simulink model "clutch_lockup"  (R2020b)
settings: Solver=ode23  StartTime=0.0  StopTime=10.0  RelTol=1e-3
model workspace (MATLAB code in the model file):
  | % Load initial conditions and other information
  | 
  | load sldemo_clutchparam;
undefined symbols (not defined in the file or in its folder): be, bv, Ie, Iv, muk, mus, R
settings Model: DataDictionary=ClutchDataDict.sldd  OrderedModelArguments=off  Creator=DELL  LastModifiedBy=DELL
settings SolverCC: MaxConsecutiveMinStep=5  ZeroCrossAlgorithm=Adaptive
settings DebuggingCC: MaxConsecutiveZCsMsg=none  IgnoredZcDiagnostic=none

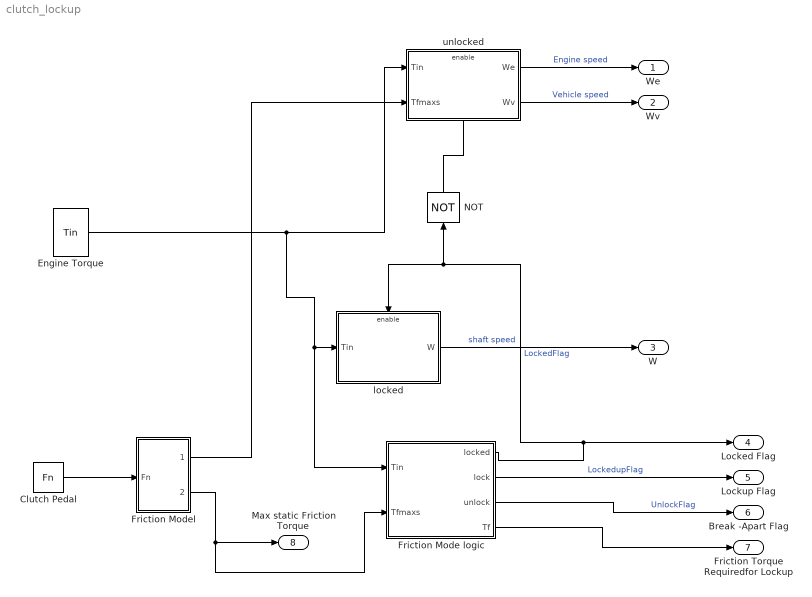
== system clutch_lockup ==
  Clutch Pedal : FromWorkspace  VariableName=Fn  ZeroCross=off
  Engine Torque : FromWorkspace  VariableName=Tin  ZeroCross=off
  Friction Mode logic : Subsystem
  Friction Model : Subsystem
  NOT : Logic  Operator=NOT  IconShape=distinctive  AllPortsSameDT=off  OutDataTypeStr=fixdt(1,16)
  locked : Subsystem
  unlocked : Subsystem
  We : Outport
  Wv : Outport  Port=2
  W : Outport  Port=3
  Locked Flag : Outport  Port=4
  Lockup Flag : Outport  Port=5
  Break -Apart Flag : Outport  Port=6
  Friction Torque Requiredfor Lockup : Outport  Port=7
  Max static Friction Torque : Outport  Port=8
  wires:
  Friction Mode logic/2(lock) -> Lockup Flag/1  "LockedupFlag"
  Friction Mode logic/1(locked) -> Locked Flag/1, NOT/1, locked/Enable  "LockedFlag"
  Friction Model/1(Tfmaxk) -> unlocked/2(Tfmaxs)
  Friction Mode logic/4(Tf) -> Friction Torque Requiredfor Lockup/1
  Friction Mode logic/3(unlock) -> Break -Apart Flag/1  "UnlockFlag"
  Friction Model/2(Tfmaxs) -> Friction Mode logic/2(Tfmaxs), Max static Friction Torque/1
  locked/1(W) -> W/1  "shaft speed"
  NOT/1 -> unlocked/Enable
  Engine Torque/1 -> unlocked/1(Tin), Friction Mode logic/1(Tin), locked/1(Tin)
  unlocked/2(Wv) -> Wv/1  "Vehicle speed"
  unlocked/1(We) -> We/1  "Engine speed"
  Clutch Pedal/1 -> Friction Model/1(Fn)

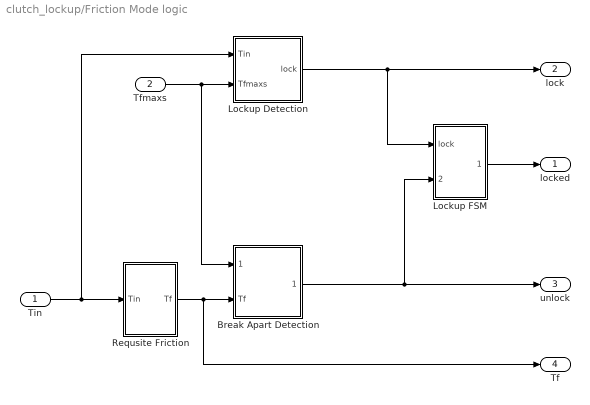
== system clutch_lockup/Friction Mode logic ==
  Tin : Inport
  Tfmaxs : Inport  Port=2
  Break Apart Detection : Subsystem
  Lockup Detection : Subsystem
  Lockup FSM : Subsystem
  Requsite Friction : Subsystem
  locked : Outport
  lock : Outport  Port=2
  unlock : Outport  Port=3
  Tf : Outport  Port=4
  wires:
  Tin/1 -> Lockup Detection/1(Tin), Requsite Friction/1(Tin)
  Requsite Friction/1(Tf) -> Tf/1, Break Apart Detection/2(Tf)
  Tfmaxs/1 -> Break Apart Detection/1(Tfmaxs), Lockup Detection/2(Tfmaxs)
  Lockup FSM/1(locked) -> locked/1
  Lockup Detection/1(lock) -> Lockup FSM/1(lock), lock/1
  Break Apart Detection/1(unlock) -> Lockup FSM/2(unlock), unlock/1

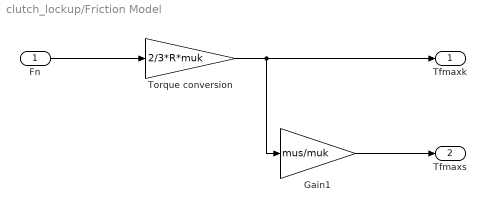
== system clutch_lockup/Friction Model ==
  Fn : Inport
  Gain1 : Gain  Gain=mus/muk
  Torque conversion : Gain  Gain=2/3*R*muk
  Tfmaxk : Outport
  Tfmaxs : Outport  Port=2
  wires:
  Fn/1 -> Torque conversion/1
  Torque conversion/1 -> Gain1/1, Tfmaxk/1
  Gain1/1 -> Tfmaxs/1

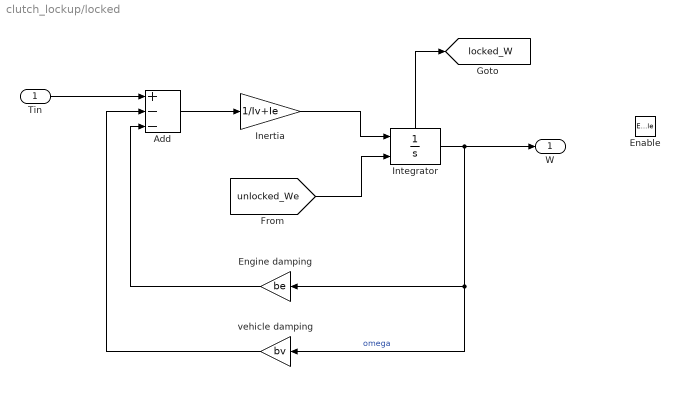
== system clutch_lockup/locked ==
  Tin : Inport
  Enable : EnablePort
  Add : Sum  Inputs=+--
  Engine damping : Gain  Gain=be
  Inertia : Gain  Gain=1/Iv+Ie
  Integrator : Integrator  InitialConditionSource=external  ShowStatePort=on
  vehicle damping : Gain  Gain=bv
  W : Outport
  tag scope: locked_W=global
  wires:
  vehicle damping/1 -> Add/2
  Integrator/1 -> W/1, Engine damping/1, vehicle damping/1  "omega"
  Tin/1 -> Add/1
  Engine damping/1 -> Add/3
  Integrator/State -> [locked_W]
  Inertia/1 -> Integrator/1
  Add/1 -> Inertia/1
  [unlocked_We] -> Integrator/2

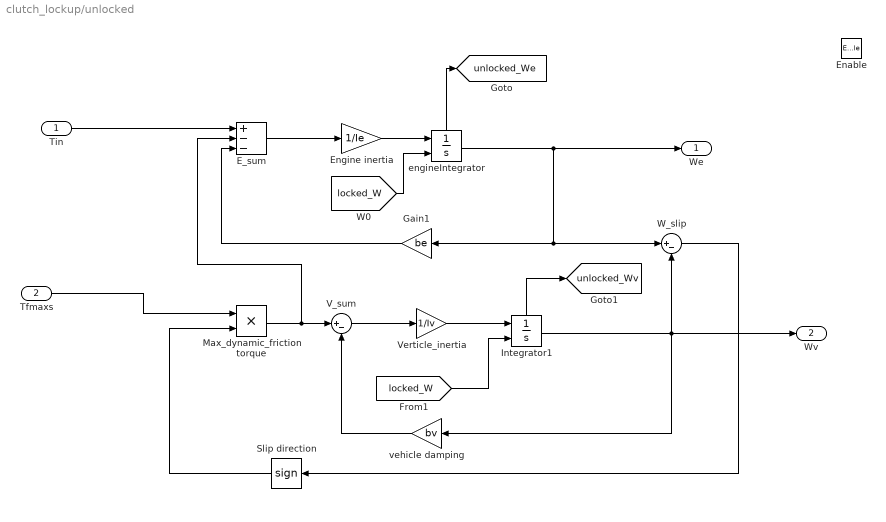
== system clutch_lockup/unlocked ==
  Tin : Inport
  Tfmaxs : Inport  Port=2
  Enable : EnablePort
  E_sum : Sum  Inputs=+--
  Engine inertia : Gain  Gain=1/Ie
  Gain1 : Gain  Gain=be
  Integrator1 : Integrator  InitialConditionSource=external  ShowStatePort=on
  Max_dynamic_friction torque : Product
  Slip direction : Signum
  V_sum : Sum  Inputs=|+-
  Verticle_inertia : Gain  Gain=1/Iv
  W_slip : Sum  Inputs=|+-
  engineIntegrator : Integrator  InitialConditionSource=external  ShowStatePort=on
  vehicle damping : Gain  Gain=bv
  We : Outport
  Wv : Outport  Port=2
  tag scope: unlocked_We=global, unlocked_Wv=global
  wires:
  Max_dynamic_friction torque/1 -> V_sum/1, E_sum/2
  E_sum/1 -> Engine inertia/1
  engineIntegrator/1 -> We/1, Gain1/1, W_slip/1
  engineIntegrator/State -> [unlocked_We]
  Integrator1/1 -> Wv/1, vehicle damping/1, W_slip/2
  Verticle_inertia/1 -> Integrator1/1
  Engine inertia/1 -> engineIntegrator/1
  [locked_W] -> engineIntegrator/2
  Slip direction/1 -> Max_dynamic_friction torque/2
  Gain1/1 -> E_sum/3
  [locked_W] -> Integrator1/2
  W_slip/1 -> Slip direction/1
  Integrator1/State -> [unlocked_Wv]
  V_sum/1 -> Verticle_inertia/1
  Tin/1 -> E_sum/1
  vehicle damping/1 -> V_sum/2
  Tfmaxs/1 -> Max_dynamic_friction torque/1

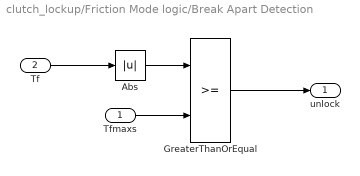
== system clutch_lockup/Friction Mode logic/Break Apart Detection ==
  Tfmaxs : Inport
  Tf : Inport  Port=2
  Abs : Abs
  GreaterThanOrEqual : RelationalOperator  OutDataTypeStr=boolean  RndMeth=Simplest
  unlock : Outport
  wires:
  Tf/1 -> Abs/1
  Tfmaxs/1 -> GreaterThanOrEqual/2
  Abs/1 -> GreaterThanOrEqual/1
  GreaterThanOrEqual/1 -> unlock/1

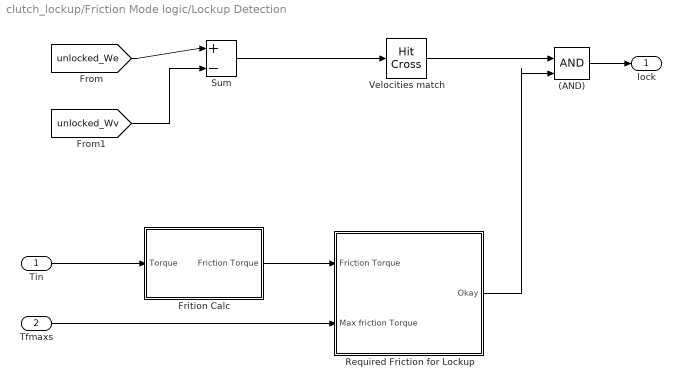
== system clutch_lockup/Friction Mode logic/Lockup Detection ==
  Tin : Inport
  Tfmaxs : Inport  Port=2
  (AND) : Logic  IconShape=distinctive  AllPortsSameDT=off  OutDataTypeStr=boolean
  Frition Calc : Subsystem
  Required Friction for Lockup : Subsystem
  Sum : Sum  Inputs=|+-
  Velocities match : HitCross
  lock : Outport
  wires:
  Tin/1 -> Frition Calc/1(Torque)
  [unlocked_We] -> Sum/1
  [unlocked_Wv] -> Sum/2
  Sum/1 -> Velocities match/1
  (AND)/1 -> lock/1
  Frition Calc/1(Friction Torque) -> Required Friction for Lockup/1(Friction Torque)
  Tfmaxs/1 -> Required Friction for Lockup/2(Max friction Torque)
  Required Friction for Lockup/1(Okay) -> (AND)/2
  Velocities match/1 -> (AND)/1

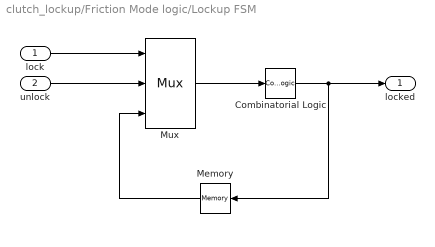
== system clutch_lockup/Friction Mode logic/Lockup FSM ==
  lock : Inport
  unlock : Inport  Port=2
  Combinatorial Logic : CombinatorialLogic  TruthTable=[0;1;0;0;1;1;1;0]
  Memory : Memory
  Mux : Mux  Inputs=3
  locked : Outport
  wires:
  lock/1 -> Mux/1
  unlock/1 -> Mux/2
  Mux/1 -> Combinatorial Logic/1
  Combinatorial Logic/1 -> Memory/1, locked/1
  Memory/1 -> Mux/3

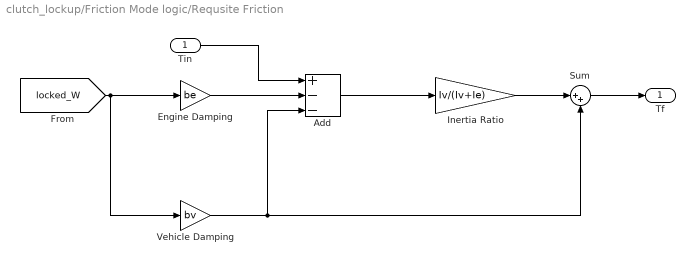
== system clutch_lockup/Friction Mode logic/Requsite Friction ==
  Tin : Inport
  Add : Sum  Inputs=+--
  Engine Damping : Gain  Gain=be
  Inertia Ratio : Gain  Gain=Iv/(Iv+Ie)
  Sum : Sum  Inputs=|++
  Vehicle Damping : Gain  Gain=bv
  Tf : Outport
  wires:
  [locked_W] -> Vehicle Damping/1, Engine Damping/1
  Engine Damping/1 -> Add/2
  Vehicle Damping/1 -> Sum/2, Add/3
  Tin/1 -> Add/1
  Add/1 -> Inertia Ratio/1
  Inertia Ratio/1 -> Sum/1
  Sum/1 -> Tf/1

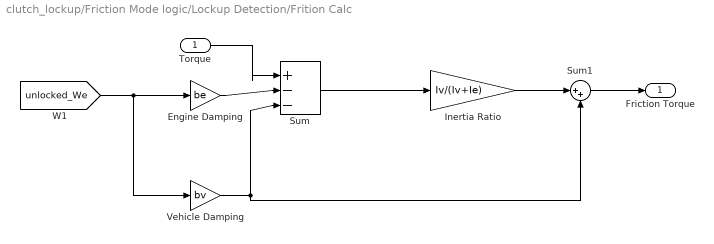
== system clutch_lockup/Friction Mode logic/Lockup Detection/Frition Calc ==
  Torque : Inport
  Engine Damping : Gain  Gain=be
  Inertia Ratio : Gain  Gain=Iv/(Iv+Ie)
  Sum : Sum  Inputs=|+--
  Sum1 : Sum  Inputs=|++
  Vehicle Damping : Gain  Gain=bv
  Friction Torque : Outport
  wires:
  [unlocked_We] -> Vehicle Damping/1, Engine Damping/1
  Engine Damping/1 -> Sum/2
  Vehicle Damping/1 -> Sum1/2, Sum/3
  Torque/1 -> Sum/1
  Sum/1 -> Inertia Ratio/1
  Inertia Ratio/1 -> Sum1/1
  Sum1/1 -> Friction Torque/1

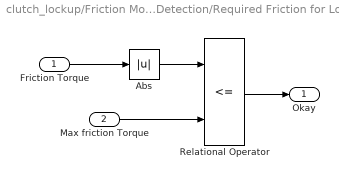
== system clutch_lockup/Friction Mode logic/Lockup Detection/Required Friction for Lockup ==
  Friction Torque : Inport
  Max friction Torque : Inport  Port=2
  Abs : Abs
  Relational Operator : RelationalOperator  Operator=<=  OutDataTypeStr=boolean  RndMeth=Simplest
  Okay : Outport
  wires:
  Friction Torque/1 -> Abs/1
  Max friction Torque/1 -> Relational Operator/2
  Abs/1 -> Relational Operator/1
  Relational Operator/1 -> Okay/1
